simulink model "LQR_pade"  (R2023b)
settings: Solver=VariableStepAuto  StartTime=0.0  StopTime=10  RelTol=1e-3
undefined symbols (not defined in the file): A, B, C, disturbance, K_tilde, kr, r
settings Model: Creator=giova  LastModifiedBy=giova

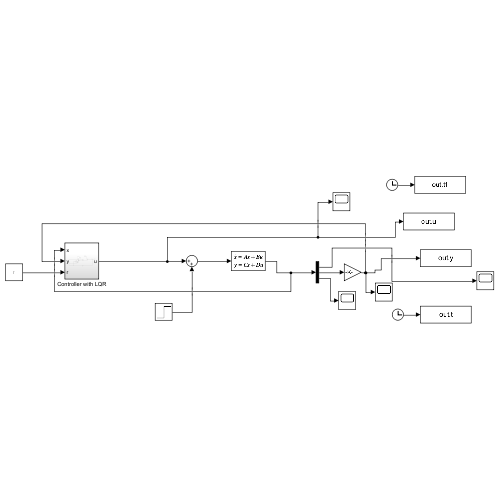
[thumbnail: Simulink's stored preview of the top-level diagram]
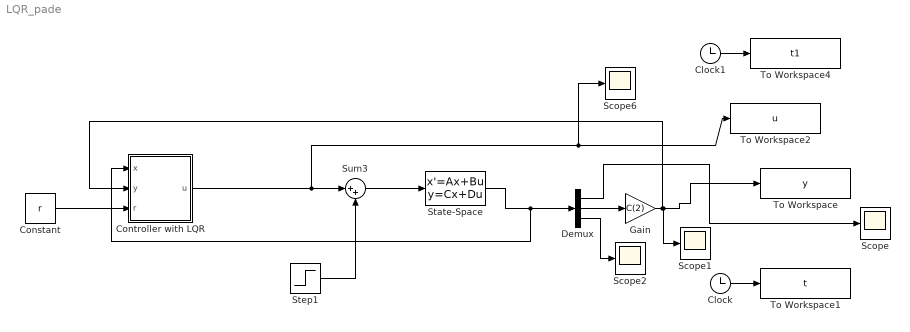
== system LQR_pade ==
  Clock : Clock
  Clock1 : Clock
  Constant : Constant  Value=r
  Controller with LQR : Subsystem
  Demux : Demux  Outputs=3
  Gain : Gain  Gain=C(2)
  Scope{,1..2,6} (4 alike) : Scope
  State-Space : StateSpace  A=A  B=B  C=eye(3)  D=[0;0;0]  InitialCondition=0
  Step1 : Step  Time=2  After=disturbance  SampleTime=0
  Sum3 : Sum  Inputs=|++
  To Workspace : ToWorkspace  VariableName=y  SampleTime=-1
  To Workspace1 : ToWorkspace  VariableName=t  SampleTime=-1
  To Workspace2 : ToWorkspace  VariableName=u  SampleTime=-1
  To Workspace4 : ToWorkspace  VariableName=t1  SampleTime=-1
  wires:
  Sum3/1 -> State-Space/1
  Controller with LQR/1(u) -> Scope6/1, To Workspace2/1, Sum3/1
  Clock/1 -> To Workspace1/1
  Demux/1 -> Scope/1
  Demux/3 -> Scope2/1
  Clock1/1 -> To Workspace4/1
  State-Space/1 -> Controller with LQR/1(x), Demux/1
  Demux/2 -> Gain/1
  Constant/1 -> Controller with LQR/3(r)
  Gain/1 -> Controller with LQR/2(y), To Workspace/1, Scope1/1
  Step1/1 -> Sum3/2

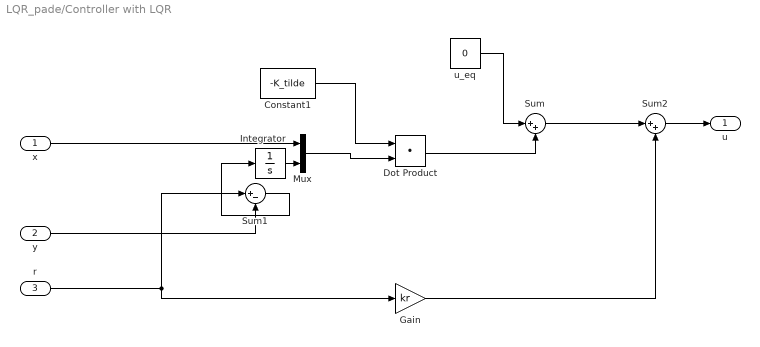
== system LQR_pade/Controller with LQR ==
  x : Inport
  y : Inport  Port=2
  r : Inport  Port=3
  Constant1 : Constant  Value=-K_tilde
  Dot Product : DotProduct  OutDataTypeStr=Inherit: Inherit via internal rule
  Gain : Gain  Gain=kr
  Integrator : Integrator
  Mux : Mux  Inputs=2
  Sum : Sum  Inputs=|++
  Sum1 : Sum  Inputs=|+-
  Sum2 : Sum  Inputs=|++
  u_eq : Constant  Value=0
  u : Outport
  wires:
  r/1 -> Sum1/1, Gain/1
  Dot Product/1 -> Sum/2
  Sum/1 -> Sum2/1
  u_eq/1 -> Sum/1
  Gain/1 -> Sum2/2
  Constant1/1 -> Dot Product/1
  Sum2/1 -> u/1
  x/1 -> Mux/1
  Mux/1 -> Dot Product/2
  y/1 -> Sum1/2
  Integrator/1 -> Mux/2
  Sum1/1 -> Integrator/1
